simulink model "soc_pmsm_cpu1_ref"  (R2023b)
settings: Solver=FixedStepAuto  StartTime=0.0  StopTime=1  RelTol=1e-3  EnableMultiTasking=on
InitFcn:
  | soc_mcb_pmsm_foc_sensorless_f28379d_data;
  | coeff = .007*Ts/50e-6;
values from neighbouring files (symbols this model uses):
  PI_params = mcb.internal.SetControllerParameters(pmsm,inverter,PU_System,T_pwm,2*Ts,Ts_speed)    [soc_mcb_pmsm_foc_sensorless_f28379d_data.m]
  pmsm = mcb_SetPMSMMotorParameters('custom')    [soc_mcb_pmsm_foc_sensorless_f28379d_data.m]
  PU_System = mcb_SetPUSystem(pmsm,inverter)    [soc_mcb_pmsm_foc_sensorless_f28379d_data.m]
  Ts = T_pwm    (= 5e-05)    [soc_mcb_pmsm_foc_sensorless_f28379d_data.m]
  Ts_speed = 10*Ts    (= 0.0005)    [soc_mcb_pmsm_foc_sensorless_f28379d_data.m]
libraries: mcbcontrolslib x4, mcbpositiondecoderlib x2, procinterlib x2, slpidlib x1
settings Model: ExtModeTrigDuration=8  Creator=The MathWorks, Inc.  LastModifiedBy=13571
settings SolverCC: AlgebraicLoopSolver=TrustRegion  PositivePriorityOrder=on
settings DataIOCC: SaveOutput=off  DSMLogging=off
settings OptimizationCC: DefaultUnderspecifiedDataType=single  EnhancedBackFolding=on  PassReuseOutputArgsAs=Individual arguments  MaxStackSize=1024  OptimizeBlockOrder=speed  DifferentSizesBufferReuse=on  OptimizationCustomize=off  DenormalBehavior=FlushToZero  EfficientTunableParamExpr=on
settings DebuggingCC: IntegerOverflowMsg=none  ParameterPrecisionLossMsg=none  ParameterTunabilityLossMsg=error  UnconnectedInputMsg=warning  UnconnectedOutputMsg=warning  UnconnectedLineMsg=warning
settings HardwareCC: ProdBitPerChar=16  ProdBitPerInt=16  ProdBitPerPointer=32  ProdBitPerSizeT=32  ProdBitPerPtrDiffT=32  ProdLargestAtomicInteger=Integer  ProdLargestAtomicFloat=None  ProdWordSize=16  ProdLongLongMode=on  ProdHWDeviceType=Texas Instruments->C2000  HardwareBoardFeatureSet=SoCBlockset
settings ModelReferenceCC: EnableRefExpFcnMdlSchedulingChecks=on  ModelReferenceNumInstancesAllowed=Single
settings SFSimCC: MATLABDynamicMemAlloc=off
settings RTWCC: Description=Embedded Coder  SystemTargetFile=ert.tlc  HardwareBoard=TI Delfino F28379D LaunchPad  TemplateMakefile=ert_default_tmf  Toolchain=Texas Instruments Code Composer Studio (C2000)  DLArmComputeVersion=19.05
settings CodeAppCC: ForceParamTrailComments=on  IgnoreCustomStorageClasses=off  OperatorAnnotations=on  SimulinkDataObjDesc=on  SFDataObjDesc=on  InsertBlockDesc=on
settings ERTTargetCC: CodeReplacementLibrary=TI C28x  ExtModeTransport=4  ExtModeStaticAlloc=on  ExtModeStaticAllocSize=10000  ExtModeMexFile=ext_xcp  ExtModeIntrfLevel=Level2 - Open

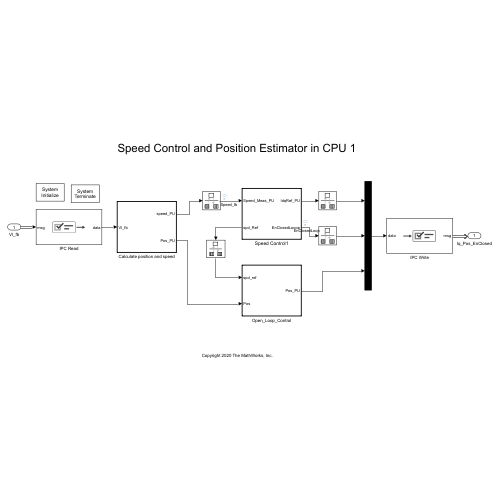
[thumbnail: Simulink's stored preview of the top-level diagram]
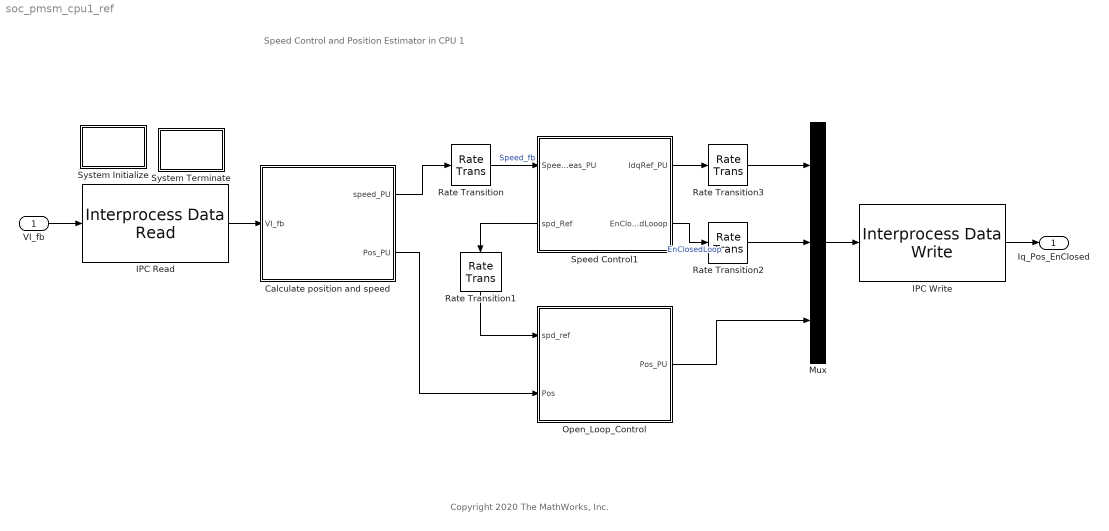
== system soc_pmsm_cpu1_ref ==
  note: Copyright 2020 The MathWorks, Inc.
  note: Speed Control and Position Estimator in CPU 1
  VI_fb : Inport  OutputPortMessageModes=m  SampleTime=Ts
  Calculate position and speed : Subsystem  TreatAsAtomicUnit=on  SystemSampleTime=Ts
  IPC Read : procinterlib/Interprocess Data Read  showPort=on  DataType=single  NumBuffers=1  DataLength=4  ChannelNum=0  IsIntEnabled=0  EnInterrupt=off  StructForBus=struct( 'signal1', uint16( 0 ), 'signal2', uint16( 0 ) )  IPCBetween=0  CurrentPU=0  PartCores=CPUx<->CPUy  SampleTime=-1  TargetType=0  ClientPU=TriCore1  ClientIntPrio=50  CurrentPUPriority=0
  IPC Write : procinterlib/Interprocess Data Write  showPort=on  ChannelNum=0  NumBuff=4  IsIntEnabled=0  EnInterrupt=off  IPCBetween=0  CurrentPU=0  DataType=uint8  PartCores=CPUx<->CPUy  TargetType=0  ClientPU=TriCore1  ClientIntPrio=50  CurrentPUPriority=0
  Mux : Mux  Inputs=3
  Open_Loop_Control : Subsystem  TreatAsAtomicUnit=on  SystemSampleTime=Ts
  Rate Transition{,1..3} (4 alike) : RateTransition  Deterministic=off
  Speed Control1 : Subsystem  TreatAsAtomicUnit=on  SystemSampleTime=Ts_speed
      settings: PortSchema="{\"entries\":[{\"content\":{\"sides\":[{\"content\":{\"connectorIds\":[\"In1\",\"Out3\"]},\"type\":\"ConnectorPlacement.EquallySpacedRectSide\",\"uuid\":\"fbea7cf5-f7a8-4f59-af6a-7947fe0f05a4\"},{\"content\":{\"connectorIds\":[\"Out1\",\"Out2\"],\"side\":\"RIGHT\"},\"type\":\"ConnectorPlacement.EquallySpacedRectSide\",\"uuid\":\"75a9dcad-2b75-4f67-a95d-e5eff8a3406e\"},{\"content\":{\"connectorIds\":[],\"side\":\"TOP\"},\"type\":\"ConnectorPlacement.EquallySpacedRectSide\",\"uuid\":\"60db082c-1dc3-46e4-b625-8ce1dcf06b1a\"},{\"content\":{\"connectorIds\":[],\"side\":\"HIDDEN\"},\"type\":\"ConnectorPlacement.EquallySpacedRectSide\",\"uuid\":\"da460418-2a03-4b9d-b669-35ae34e5ace8\"}]},\"type\":\"ConnectorPlacement.EquallySpacedConnector\",\"uuid\":\"a08698bb-f2a0-42fa-b2bd-4751e83f662c\"}],\"packageUris\":[\"http://schema.mathworks.com/mf0/Connector/R2020b\"],\"version\":\"1.0\"}"
  System Initialize : Subsystem  mask(System Initialize){ShowInLibBrowser=0}
      mask prompts: ShowInLibBrowser "Simulink:masks:CustCodeMaskParam1_MP"
      settings: CopyFcn=cccopyfcn(gcb)  OpenFcn=ccopenfcn('System Initialize Function')
      mask Help: eval('feval(''rtwprivate'',''rtwhelpview'',''rtw_sys_initialize_block'')');
      mask Display: disp('System\nInitialize');
  System Terminate : Subsystem  mask(System Terminate){ShowInLibBrowser=0}
      mask prompts: ShowInLibBrowser "Simulink:masks:CustCodeMaskParam1_MP"
      settings: CopyFcn=cccopyfcn(gcb)  OpenFcn=ccopenfcn('System Terminate Function')
      mask Help: eval('feval(''rtwprivate'',''rtwhelpview'',''rtw_sys_terminate_block'')');
      mask Display: disp('System\nTerminate');
  Iq_Pos_EnClosed : Outport  InputPortMessageModes=m  InitialOutput=0  VectorParamsAs1DForOutWhenUnconnected=off
  wires:
  Open_Loop_Control/1(Pos_PU) -> Mux/3
  Calculate position and speed/2(Pos_PU) -> Open_Loop_Control/2(Pos)
  Calculate position and speed/1(speed_PU) -> Rate Transition/1
  Rate Transition1/1 -> Open_Loop_Control/1(spd_ref)
  Rate Transition3/1 -> Mux/1
  IPC Write/1 -> Iq_Pos_EnClosed/1
  VI_fb/1 -> IPC Read/1
  IPC Read/1 -> Calculate position and speed/1(VI_fb)
  Rate Transition/1 -> Speed Control1/1(Speed_Meas_PU)  "Speed_fb"
  Mux/1 -> IPC Write/1
  Speed Control1/3(spd_Ref) -> Rate Transition1/1
  Speed Control1/1(IdqRef_PU) -> Rate Transition3/1
  Speed Control1/2(EnClosedLooop) -> Rate Transition2/1  "EnClosedLoop"
  Rate Transition2/1 -> Mux/2

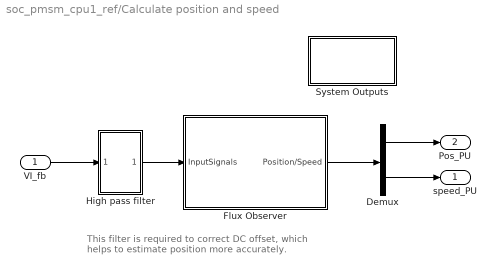
== system soc_pmsm_cpu1_ref/Calculate position and speed ==
  note: This filter is required to correct DC offset,
      | which helps to estimate position more accurately.
  VI_fb : Inport
  Demux : Demux  Outputs=2
  Flux Observer : Subsystem
  High pass filter : Subsystem
  System Outputs : Subsystem  mask(System Outputs){ShowInLibBrowser=0}
      mask prompts: ShowInLibBrowser "Simulink:masks:CustCodeMaskParam1_MP"
      settings: CopyFcn=cccopyfcn(gcb)  OpenFcn=ccopenfcn('System Outputs Function')
      mask Help: eval('feval(''rtwprivate'',''rtwhelpview'',''rtw_sys_outputs_block'')');
      mask Display: disp('System\nOutputs');
  speed_PU : Outport
  Pos_PU : Outport  Port=2
  wires:
  Demux/1 -> Pos_PU/1
  Demux/2 -> speed_PU/1
  Flux Observer/1(Position/Speed) -> Demux/1
  VI_fb/1 -> High pass filter/1(In1)
  High pass filter/1(Out1) -> Flux Observer/1(InputSignals)

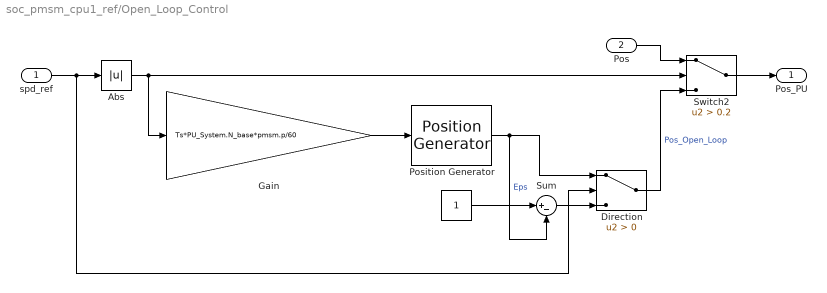
== system soc_pmsm_cpu1_ref/Open_Loop_Control ==
  spd_ref : Inport
  Pos : Inport  Port=2
  " " : Constant  OutDataTypeStr=dataType  SampleTime=-1
  Abs : Abs  SaturateOnIntegerOverflow=off
  Direction : Switch  Criteria=u2 > Threshold  OutDataTypeStr=dataType  RndMeth=Simplest  SaturateOnIntegerOverflow=off  InputSameDT=off
  Gain : Gain  Gain=Ts*PU_System.N_base*pmsm.p/60  OutDataTypeStr=Inherit: Same as input  ParamDataTypeStr=Inherit: Same as input
  Position Generator : mcbcontrolslib/Position Generator  AngleOutput=Per-unit  ExternalReset=none  Offset=0
  Sum : Sum  Inputs=|+-  RndMeth=Simplest  OutDataTypeStr=Inherit: Same as first input
  Switch2 : Switch  Criteria=u2 > Threshold  Threshold=0.2  SaturateOnIntegerOverflow=off  InputSameDT=off
  Pos_PU : Outport
  wires:
  Sum/1 -> Direction/3
  Switch2/1 -> Pos_PU/1
  Pos/1 -> Switch2/1
  " "/1 -> Sum/1
  Direction/1 -> Switch2/3  "Pos_Open_Loop"
  Gain/1 -> Position Generator/1
  spd_ref/1 -> Abs/1, Direction/2
  Position Generator/1 -> Direction/1, Sum/2  "Eps"
  Abs/1 -> Switch2/2, Gain/1

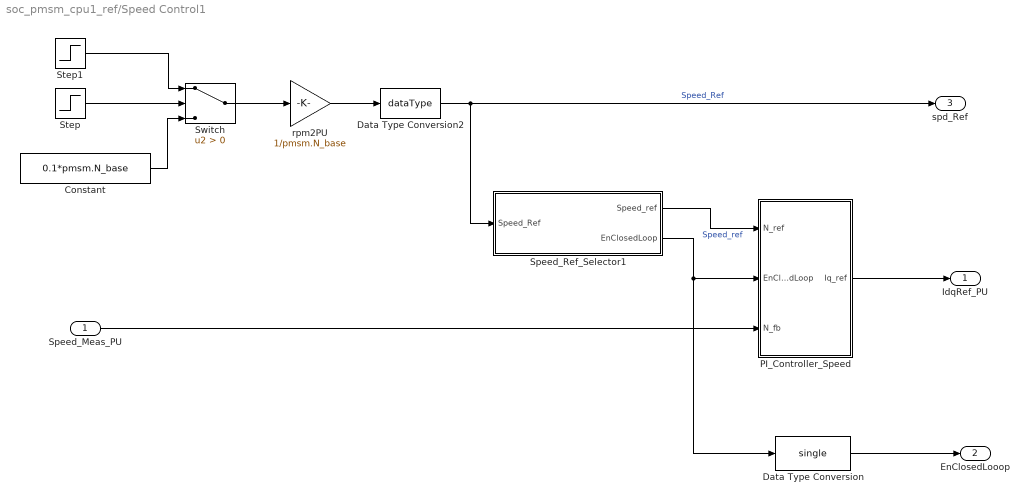
== system soc_pmsm_cpu1_ref/Speed Control1 ==
  Speed_Meas_PU : Inport
  Constant : Constant  Value=0.1*pmsm.N_base  SampleTime=-1
  Data Type Conversion : DataTypeConversion  OutDataTypeStr=single  RndMeth=Simplest  SaturateOnIntegerOverflow=off
  Data Type Conversion2 : DataTypeConversion  OutDataTypeStr=dataType  RndMeth=Simplest  SaturateOnIntegerOverflow=off
  PI_Controller_Speed : Subsystem
  Speed_Ref_Selector1 : Subsystem
  Step : Step  Time=.05
  Step1 : Step  Time=.3  Before=0.5*pmsm.N_base  After=0.7*pmsm.N_base
  Switch : Switch  Criteria=u2 > Threshold  SaturateOnIntegerOverflow=off  InputSameDT=off
  rpm2PU : Gain  Gain=1/pmsm.N_base  RndMeth=Simplest  OutDataTypeStr=Inherit: Same as input
  IdqRef_PU : Outport  VectorParamsAs1DForOutWhenUnconnected=off
  EnClosedLooop : Outport  Port=2
  spd_Ref : Outport  Port=3  VectorParamsAs1DForOutWhenUnconnected=off
  wires:
  Speed_Meas_PU/1 -> PI_Controller_Speed/3(N_fb)
  Data Type Conversion2/1 -> Speed_Ref_Selector1/1(Speed_Ref), spd_Ref/1  "Speed_Ref"
  rpm2PU/1 -> Data Type Conversion2/1
  Speed_Ref_Selector1/1(Speed_ref) -> PI_Controller_Speed/1(N_ref)  "Speed_ref"
  Speed_Ref_Selector1/2(EnClosedLoop) -> PI_Controller_Speed/2(EnClosedLoop), Data Type Conversion/1
  PI_Controller_Speed/1(Iq_ref) -> IdqRef_PU/1
  Data Type Conversion/1 -> EnClosedLooop/1
  Step1/1 -> Switch/1
  Step/1 -> Switch/2
  Constant/1 -> Switch/3
  Switch/1 -> rpm2PU/1

== system soc_pmsm_cpu1_ref/System Initialize ==

== system soc_pmsm_cpu1_ref/System Terminate ==

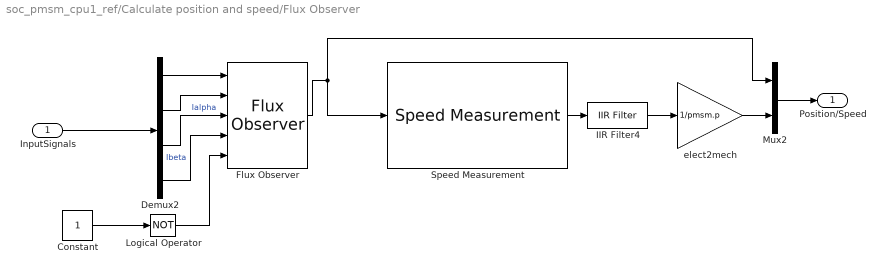
== system soc_pmsm_cpu1_ref/Calculate position and speed/Flux Observer ==
  InputSignals : Inport
  Constant : Constant  SampleTime=-1
  Demux2 : Demux
  Flux Observer : mcbpositiondecoderlib/Flux Observer  MotorSelection=PMSM  DataTypeSelect=off  BlockInputUnit=Per-unit  PerUnitVoltage=PU_System.V_base  PerUnitCurrent=PU_System.I_base  PositionSelect=on  FluxSelect=off  TorqueSelect=off  PolePairs=4  StatorResistance=pmsm.Rs  StatorDAxisInductance=pmsm.Ld  StatorLeakageInductance=0.0068  RotorLeakageInductance=0.0068  MagnetizingInductance=0.0300  CutoffFreq=3.1863  BlockSampleTime=Ts  PositionUnit=Per-unit  PositionDatatype=dataType  FluxUnit=Weber  PerUnitFlux=0.1  FluxDatatype=single  TorqueUnit=Nm  PerUnitTorque=100  TorqueDatatype=single  DataType=0
  IIR Filter4 : mcbcontrolslib/IIR Filter  VariantControl=Low Pass Filter  VariantSelect=Low-pass  Filter_constant=.01  advancedSettings=off  Ts=50e-6  cutOff_freq=32.1525
  Logical Operator : Logic  Operator=NOT  IconShape=distinctive  AllPortsSameDT=off  OutDataTypeStr=boolean
  Mux2 : Mux  Inputs=2
  Speed Measurement : mcbpositiondecoderlib/Speed Measurement  PositionUnit=Per unit  PositionScalingDatatype=uint32  SpeedCalculationMode=Time interval for speed calculation  SampleTimeAsync=Ts  MaximumApplicationSpeed=60000  SpeedResolution=5e-6  DelayLength=10  MaximumMeasurableSpeed=59999  MeasurableSpeedResolution=2.794e-05  SpeedUnit=Per unit based on dialog  PerUnitSpeed=PU_System.N_base  SpeedDataType=dataType
  elect2mech : Gain  Gain=1/pmsm.p  RndMeth=Simplest  OutDataTypeStr=Inherit: Same as input
  Position/Speed : Outport
  wires:
  InputSignals/1 -> Demux2/1
  Demux2/1 -> Flux Observer/1
  Demux2/2 -> Flux Observer/2
  Mux2/1 -> Position/Speed/1
  Speed Measurement/1 -> IIR Filter4/1
  elect2mech/1 -> Mux2/2
  Demux2/3 -> Flux Observer/3  "Ialpha"
  Demux2/4 -> Flux Observer/4  "Ibeta"
  IIR Filter4/1 -> elect2mech/1
  Flux Observer/1 -> Speed Measurement/1, Mux2/1
  Logical Operator/1 -> Flux Observer/5
  Constant/1 -> Logical Operator/1

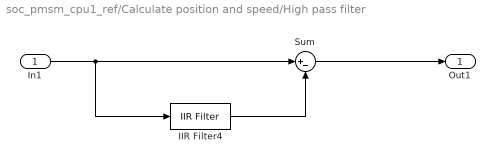
== system soc_pmsm_cpu1_ref/Calculate position and speed/High pass filter ==
  In1 : Inport
  IIR Filter4 : mcbcontrolslib/IIR Filter  VariantControl=Low Pass Filter  VariantSelect=Low-pass  Filter_constant=coeff  advancedSettings=off  Ts=50e-6  cutOff_freq=1
  Sum : Sum  Inputs=|+-  RndMeth=Simplest
  Out1 : Outport
  wires:
  IIR Filter4/1 -> Sum/2
  In1/1 -> Sum/1, IIR Filter4/1
  Sum/1 -> Out1/1

== system soc_pmsm_cpu1_ref/Calculate position and speed/System Outputs ==

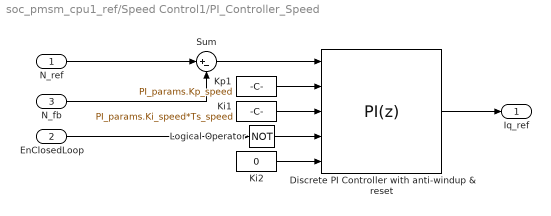
== system soc_pmsm_cpu1_ref/Speed Control1/PI_Controller_Speed ==
  N_ref : Inport
  EnClosedLoop : Inport  Port=2
  N_fb : Inport  Port=3
  Discrete PI Controller with anti-windup & reset : slpidlib/PID Controller  Controller=PI  Form=Parallel  TimeDomain=Discrete-time  UseExternalTs=off  SampleTime=-1  IntegratorMethod=Forward Euler  FilterMethod=Forward Euler  ControllerParametersSource=external  P=1  I=1  UseKiTs=on  D=0  N=100  UseFilter=on  TunerSelectOption=Transfer Function Based (PID Tuner App)  InitialConditionSource=external  InitialConditionForIntegrator=0  InitialConditionForFilter=0  DifferentiatorICPrevScaledInput=0  ExternalReset=level  TrackingMode=off  Kt=1  LimitOutput=on  SatLimitsSource=internal  UpperSaturationLimit=1  LowerSaturationLimit=-1  LinearizeAsGain=on  AntiWindupMode=clamping  Kb=1  LimitIntegrator=off  UpperIntegratorSaturationLimit=inf  LowerIntegratorSaturationLimit=-inf  RndMeth=Simplest  POutMin=[]  POutMax=[]  IOutMin=[]  IOutMax=[]  DOutMin=[]  DOutMax=[]  NOutMin=[]  NOutMax=[]  SumOutMin=[]  SumOutMax=[]  SaturationOutDataTypeStr=Inherit: Inherit via back propagation  SaturationOutMin=[]  SaturationOutMax=[]  PParamMin=[]  PParamMax=[]  IParamMin=[]  IParamMax=[]  DParamMin=[]  DParamMax=[]  NParamMin=[]  NParamMax=[]  KbParamMin=[]  KbParamMax=[]  KtParamMin=[]  KtParamMax=[]  KbOutMin=[]  KbOutMax=[]  KtOutMin=[]  KtOutMax=[]  IntegratorOutMin=[]  IntegratorOutMax=[]  FilterOutMin=[]  FilterOutMax=[]  SumI1OutMin=[]  SumI1OutMax=[]  SumI2OutMin=[]  SumI2OutMax=[]  SumI3OutMin=[]  SumI3OutMax=[]  SumI4OutMin=[]  SumI4OutMax=[]  SumDOutMin=[]  SumDOutMax=[]  DifferentiatorOutMin=[]  DifferentiatorOutMax=[]  FilterDiffOutCoefMin=[]  FilterDiffOutCoefMax=[]  ReciprocalOutMin=[]  ReciprocalOutMax=[]  SumDenOutMin=[]  SumDenOutMax=[]  SumNumOutMin=[]  SumNumOutMax=[]  DivideOutMin=[]  DivideOutMax=[]  UdiffTsProdOutMin=[]  UdiffTsProdOutMax=[]  NTsProdOutMin=[]  NTsProdOutMax=[]  UintegralTsProdOutMin=[]  UintegralTsProdOutMax=[]  UngainTsProdOutMin=[]  UngainTsProdOutMax=[]  ClampingZeroOutDataTypeStr=Inherit: Inherit via back propagation  ClampingZeroOutMin=[]  ClampingZeroOutMax=[]  FilterDenConstantOutDataTypeStr=Inherit: Inherit via back propagation  FilterDenConstantOutMin=[]  FilterDenConstantOutMax=[]  PCopyOutDataTypeStr=Inherit: Inherit via back propagation  PCopyOutMin=[]  PCopyOutMax=[]  NCopyOutDataTypeStr=Inherit: Inherit via back propagation  NCopyOutMin=[]  NCopyOutMax=[]  IntegratorContinuousStateAttributes=''  IntegratorStateMustResolveToSignalObject=off  IntegratorRTWStateStorageClass=Auto  FilterContinuousStateAttributes=''  FilterStateMustResolveToSignalObject=off  FilterRTWStateStorageClass=Auto  ParallelPVariant=ExternalParameters  IdealPVariant=Disabled  IVariant=ExternalParameters  DVariant=Disabled  IntegratorVariant=Discrete  SatVariant=Enabled  AWVariant=DiscClampingParallel  PCopyVariant=Disabled  TRVariant=Disabled  FdbkBlocksVariant=Forward  IdealPFdbkVariant=Disabled  SatFdbkVariant=Disabled  DerivativeFilterVariant=Disabled  NVariant=Disabled  NCopyVariant=Disabled_SignalSpec  FilterICVariant=Disabled  IntegratorICVariant=ExternalICs  ExternalResetVariant=ExternalReset  TRSumVariant=Passthrough  SumFdbkVariant=Disabled  SumVariant=Sum_PI  TsampFilterVariant=InternalTs  TsampNgainVariant=Passthrough  TsampIntegralVariant=Disabled_SignalSpec  ExternalSaturationOutDataTypeStr=Inherit: Same as second input
      settings: LibrarySourceBlock=mcbcontrolslib/PI Controller
  Ki1 : Constant  Value=PI_params.Ki_speed*Ts_speed  OutDataTypeStr=dataType  SampleTime=-1
  Ki2 : Constant  Value=0  OutDataTypeStr=dataType  SampleTime=-1
  Kp1 : Constant  Value=PI_params.Kp_speed  OutDataTypeStr=dataType  SampleTime=-1
  Logical Operator : Logic  Operator=NOT  IconShape=distinctive  AllPortsSameDT=off  OutDataTypeStr=boolean
  Sum : Sum  Inputs=|+-  OutDataTypeStr=Inherit: Same as first input
  Iq_ref : Outport  VectorParamsAs1DForOutWhenUnconnected=off
  wires:
  Discrete PI Controller with anti-windup & reset/1 -> Iq_ref/1
  Ki1/1 -> Discrete PI Controller with anti-windup & reset/3
  Kp1/1 -> Discrete PI Controller with anti-windup & reset/2
  N_fb/1 -> Sum/2
  N_ref/1 -> Sum/1
  Sum/1 -> Discrete PI Controller with anti-windup & reset/1
  Logical Operator/1 -> Discrete PI Controller with anti-windup & reset/4
  Ki2/1 -> Discrete PI Controller with anti-windup & reset/5
  EnClosedLoop/1 -> Logical Operator/1

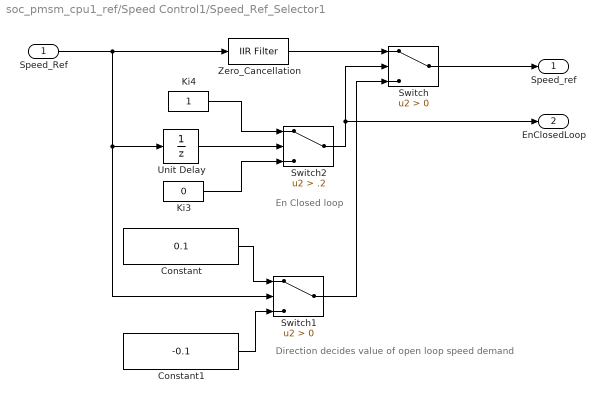
== system soc_pmsm_cpu1_ref/Speed Control1/Speed_Ref_Selector1 ==
  note: Direction decides value of open loop speed demand
  note: En Closed loop
  Speed_Ref : Inport
  Constant : Constant  Value=0.1  OutDataTypeStr=dataType
  Constant1 : Constant  Value=-0.1  OutDataTypeStr=dataType
  Ki3 : Constant  Value=0  OutDataTypeStr=dataType  SampleTime=-1
  Ki4 : Constant  OutDataTypeStr=dataType  SampleTime=-1
  Switch : Switch  Criteria=u2 > Threshold  SaturateOnIntegerOverflow=off  InputSameDT=off
  Switch1 : Switch  Criteria=u2 > Threshold  SaturateOnIntegerOverflow=off  InputSameDT=off
  Switch2 : Switch  Criteria=u2 > Threshold  Threshold=.2  SaturateOnIntegerOverflow=off  InputSameDT=off
  Unit Delay : UnitDelay  SampleTime=-1  HasFrameUpgradeWarning=on
  Zero_Cancellation : mcbcontrolslib/IIR Filter  VariantControl=Low Pass Filter  VariantSelect=Low-pass  Filter_constant=.01*(Ts_speed/Ts)  advancedSettings=off  Ts=50e-6  cutOff_freq=1
  Speed_ref : Outport
  EnClosedLoop : Outport  Port=2
  wires:
  Switch1/1 -> Switch/3
  Constant/1 -> Switch1/1
  Speed_Ref/1 -> Unit Delay/1, Switch1/2, Zero_Cancellation/1
  Switch2/1 -> EnClosedLoop/1, Switch/2
  Constant1/1 -> Switch1/3
  Switch/1 -> Speed_ref/1
  Ki3/1 -> Switch2/3
  Ki4/1 -> Switch2/1
  Unit Delay/1 -> Switch2/2
  Zero_Cancellation/1 -> Switch/1
